simulink model "R19_Modelo_lineal_c_2GDL_2021"  (R2019a)
settings: Solver=VariableStepAuto  StartTime=0.0  StopTime=0.1  RelTol=1e-3
undefined symbols (not defined in the file): Ac, Bc, Cc, Dc, initial_conds, pod, z_0, z_lev
libraries: shared3dof x1, libH7_3DOF x1
settings Model: Creator=EDMAOR  LastModifiedBy=emate

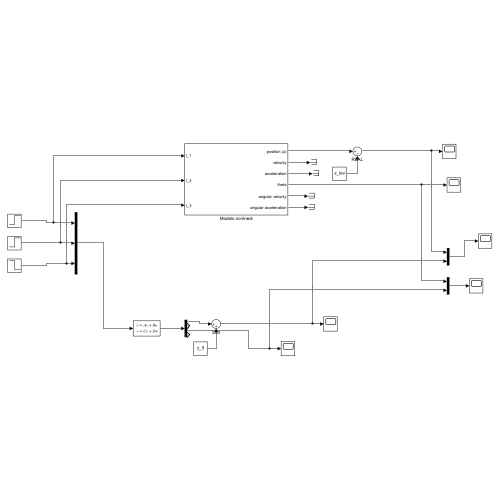
[thumbnail: Simulink's stored preview of the top-level diagram]
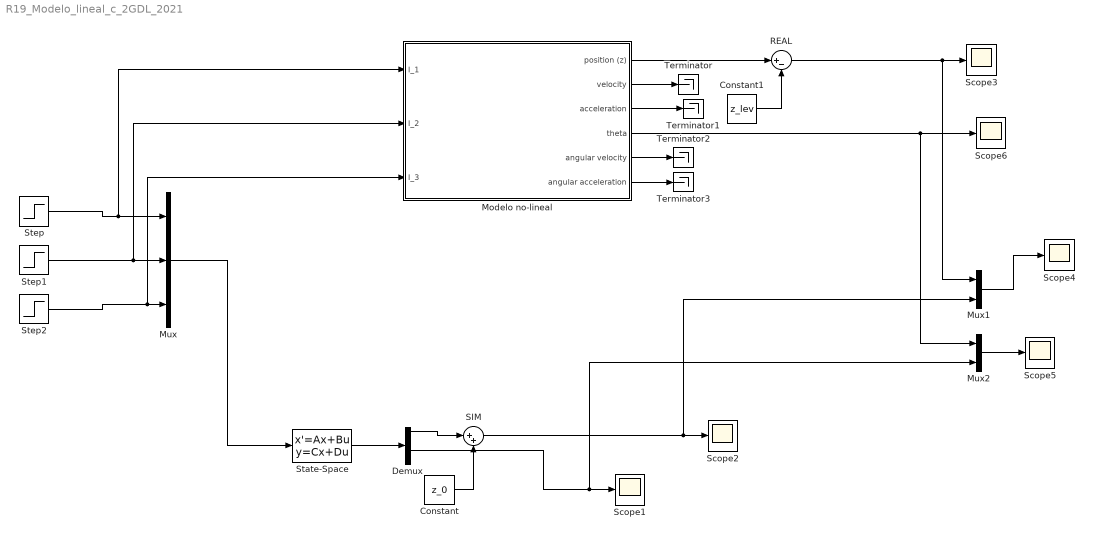
== system R19_Modelo_lineal_c_2GDL_2021 ==
  Constant : Constant  Value=z_0
  Constant1 : Constant  Value=z_lev
  Demux : Demux
  Modelo no-lineal : Subsystem
  Mux : Mux  Inputs=3
  Mux1 : Mux  Inputs=2
  Mux2 : Mux  Inputs=2
  REAL : Sum  Inputs=|+-
  SIM : Sum  Inputs=|++
  Scope{1..6} (6 alike) : Scope
  State-Space : StateSpace  A=Ac  B=Bc  C=Cc  D=Dc  InitialCondition=[0 0 0 0]
  Step : Step  Time=0  After=10  SampleTime=0
  Step1 : Step  Time=0  After=10  SampleTime=0
  Step2 : Step  Time=0  After=-10  SampleTime=0
  Terminator{,1..3} (4 alike) : Terminator
  wires:
  Constant/1 -> SIM/2
  Demux/1 -> SIM/1
  State-Space/1 -> Demux/1
  SIM/1 -> Mux1/2, Scope2/1
  Step/1 -> Modelo no-lineal/1(I_1), Mux/1
  Step1/1 -> Modelo no-lineal/2(I_2), Mux/2
  Step2/1 -> Modelo no-lineal/3(I_3), Mux/3
  Mux/1 -> State-Space/1
  Demux/3 -> Mux2/2, Scope1/1
  Mux1/1 -> Scope4/1
  Mux2/1 -> Scope5/1
  Modelo no-lineal/2(velocity) -> Terminator/1
  Modelo no-lineal/3(acceleration) -> Terminator1/1
  Modelo no-lineal/4(theta) -> Mux2/1, Scope6/1
  Modelo no-lineal/5(angular velocity) -> Terminator2/1
  Modelo no-lineal/6(angular acceleration) -> Terminator3/1
  Modelo no-lineal/1(position (z)) -> REAL/1
  REAL/1 -> Mux1/1, Scope3/1
  Constant1/1 -> REAL/2

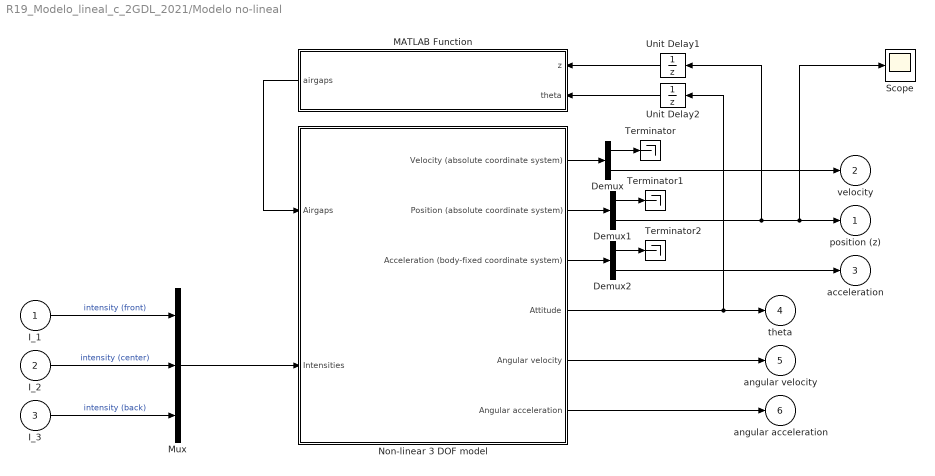
== system R19_Modelo_lineal_c_2GDL_2021/Modelo no-lineal ==
  I_1 : Inport
  I_2 : Inport  Port=2
  I_3 : Inport  Port=3
  Demux : Demux  Outputs=2
  Demux1 : Demux  Outputs=2
  Demux2 : Demux  Outputs=2
  MATLAB Function : MATLAB Function  TreatAsAtomicUnit=on
  Mux : Mux  Inputs=3
  Non-linear 3 DOF model : Subsystem  AncestorBlock=libH7_3DOF/Non-linear 3 DOF model
  Scope : Scope
  Terminator : Terminator
  Terminator1 : Terminator
  Terminator2 : Terminator
  Unit Delay1 : UnitDelay  InitialCondition=initial_conds.x_0(3)  SampleTime=-1  HasFrameUpgradeWarning=on
  Unit Delay2 : UnitDelay  SampleTime=-1  HasFrameUpgradeWarning=on
  position (z) : Outport
  velocity : Outport  Port=2
  acceleration : Outport  Port=3
  theta : Outport  Port=4
  angular velocity : Outport  Port=5
  angular acceleration : Outport  Port=6
  wires:
  Mux/1 -> Non-linear 3 DOF model/2(Intensities)
  I_1/1 -> Mux/1  "intensity (front)"
  I_2/1 -> Mux/2  "intensity (center)"
  I_3/1 -> Mux/3  "intensity (back)"
  Non-linear 3 DOF model/4("Attitude ") -> theta/1, Unit Delay2/1
  Non-linear 3 DOF model/5(Angular velocity) -> angular velocity/1
  Non-linear 3 DOF model/1(Velocity (absolute coordinate system)) -> Demux/1
  Demux/1 -> Terminator/1
  Demux/2 -> velocity/1
  Demux1/1 -> Terminator1/1
  Demux1/2 -> Unit Delay1/1, Scope/1, position (z)/1
  Non-linear 3 DOF model/2(Position (absolute coordinate system)) -> Demux1/1
  Demux2/1 -> Terminator2/1
  Demux2/2 -> acceleration/1
  Non-linear 3 DOF model/3(Acceleration (body-fixed coordinate system)) -> Demux2/1
  Unit Delay1/1 -> MATLAB Function/1(z)
  Unit Delay2/1 -> MATLAB Function/2(theta)
  MATLAB Function/1(airgaps) -> Non-linear 3 DOF model/1(Airgaps)
  Non-linear 3 DOF model/6(Angular acceleration) -> angular acceleration/1

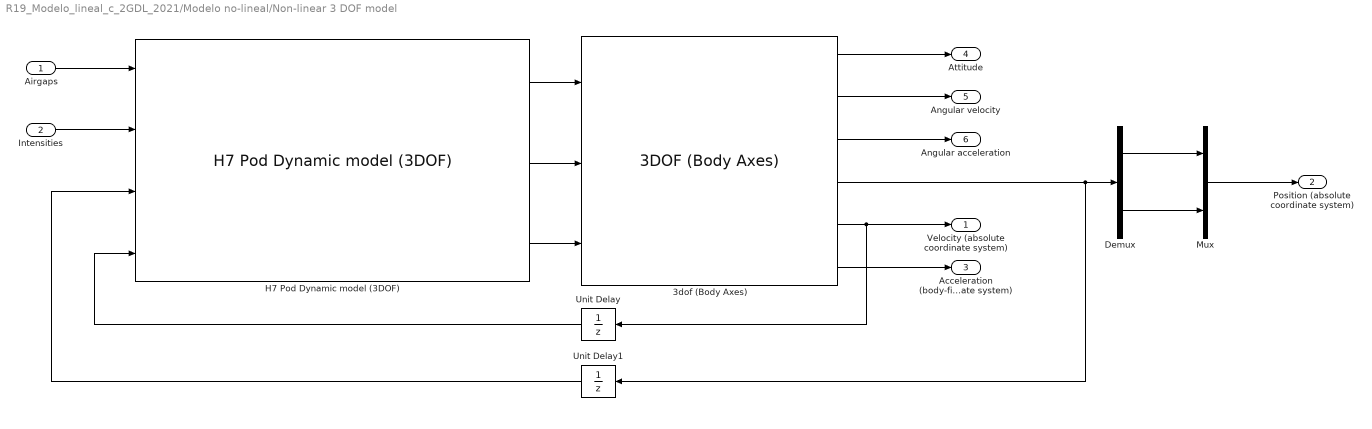
== system R19_Modelo_lineal_c_2GDL_2021/Modelo no-lineal/Non-linear 3 DOF model ==
  Airgaps : Inport
  Intensities : Inport  Port=2
  3dof (Body Axes) : shared3dof/3DOF (Body Axes)  units=Metric (MKS)  mtype=Fixed  v_ini=1e-10  theta_ini=initial_conds.ang_0(2)  alpha_ini=0  pos_ini=initial_conds.x_0(1:2:3)  q_ini=initial_conds.w_0(2)  mass=pod.mass.mass  mass_e=0.5  mass_f=3.0  Iyy=pod.mass.inertia(2,2)  Iyy_e=0.5  Iyy_f=3.0  g_in=Internal  g=9.81  vre_flag=off  abi_flag=off  aMode=0  vel_statename=''  theta_statename=''  pos_statename=''  q_statename=''  mass_statename=''
      settings: SourceProductBaseCode=AE,PW,DR,MT,UV,VE
  Demux : Demux  Outputs=2
  H7 Pod Dynamic model (3DOF) : libH7_3DOF/H7 Pod Dynamic model (3DOF)  SystemSampleTime=-1  Latency=0  AutoFrameSizeCalculation=off
      settings: SourceProductName=00. H7 Pod models
  Mux : Mux  Inputs=2
  Unit Delay : UnitDelay  InitialCondition=[0,0]  SampleTime=-1  HasFrameUpgradeWarning=on
  Unit Delay1 : UnitDelay  InitialCondition=initial_conds.x_0(1:2:3)  SampleTime=-1  HasFrameUpgradeWarning=on
  Velocity (absolute coordinate system) : Outport
  Position (absolute coordinate system) : Outport  Port=2
  Acceleration (body-fixed coordinate system) : Outport  Port=3
  "Attitude " : Outport  Port=4
  Angular velocity : Outport  Port=5
  Angular acceleration : Outport  Port=6
  wires:
  Demux/2 -> Mux/2
  Demux/1 -> Mux/1
  Unit Delay1/1 -> H7 Pod Dynamic model (3DOF)/3
  Unit Delay/1 -> H7 Pod Dynamic model (3DOF)/4
  Mux/1 -> Position (absolute coordinate system)/1
  3dof (Body Axes)/1 -> "Attitude "/1
  3dof (Body Axes)/4 -> Unit Delay1/1, Demux/1
  3dof (Body Axes)/5 -> Unit Delay/1, Velocity (absolute coordinate system)/1
  3dof (Body Axes)/3 -> Angular acceleration/1
  3dof (Body Axes)/6 -> Acceleration (body-fixed coordinate system)/1
  Airgaps/1 -> H7 Pod Dynamic model (3DOF)/1
  Intensities/1 -> H7 Pod Dynamic model (3DOF)/2
  H7 Pod Dynamic model (3DOF)/2 -> 3dof (Body Axes)/2
  H7 Pod Dynamic model (3DOF)/3 -> 3dof (Body Axes)/3
  3dof (Body Axes)/2 -> Angular velocity/1
  H7 Pod Dynamic model (3DOF)/1 -> 3dof (Body Axes)/1

== matlab function R19_Modelo_lineal_c_2GDL_2021/Modelo no-lineal/MATLAB Function ==
  data: z input; theta input; airgaps output; pod parameter
function airgaps = pos2ag2D(z, theta, pod)
% Computes the airgaps (mm) as a function of the position (m) and 
% attitude (rad) of the prototype
% ═════════════════════════════════════════════════════════════════════════
% Last updated: 15.01.2022
% ═════════════════════════════════════════════════════════════════════════

airgaps = zeros(3,1);

airgaps(1) = z - pod.geometry.x_LEV * sin(theta) - pod.geometry.z_LEV * cos(theta);
airgaps(2) = z                                   - pod.geometry.z_LEV * cos(theta);
airgaps(3) = z + pod.geometry.x_LEV * sin(theta) - pod.geometry.z_LEV * cos(theta);

airgaps = airgaps * 1e3;

%if any(airgaps<=11)
%    airgaps = 11 * ones(3,1);
%elseif any(airgaps>=23)
%    airgaps = 23 * ones(3,1);
end
